simulink model "two_mass_sys"  (R2013b)
settings: Solver=ode45  StartTime=0.0  StopTime=10.0  RelTol=1e-3
undefined symbols (not defined in the file): Cw, JL, Jm, Ks
libraries: powerlib x1
settings Model: Creator=User  LastModifiedBy=User

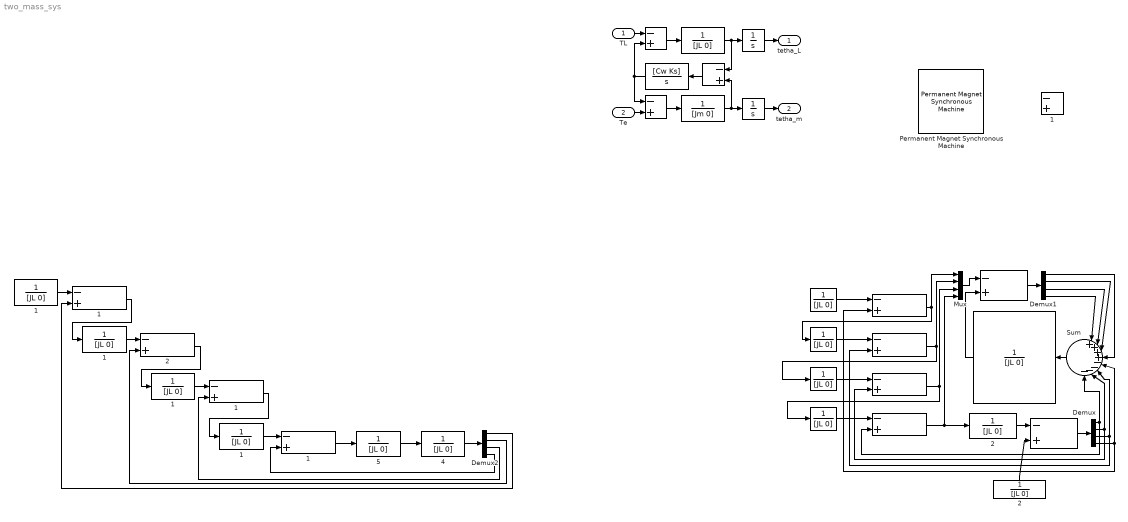
== system two_mass_sys ==
  TL : Inport
  Te : Inport  Port=2
  " " : TransferFcn  Numerator=[Cw Ks]  Denominator=[1 0]
    {,2,4..5} (4 alike) : TransferFcn  Denominator=[JL 0]
  "   " : TransferFcn  Denominator=[Jm 0]
  "    " : Integrator
  "     " : Integrator
  "       " : TransferFcn  Denominator=[JL 0]
  "        " : Sum  Inputs=-+
  "         " : Sum  Inputs=-+
  "           " : Sum  Inputs=-+
  "            " : Sum  Inputs=-+
  "              " : TransferFcn  Denominator=[JL 0]
  "                " : Sum  Inputs=-+
  "                      " : TransferFcn  Denominator=[JL 0]
  "                        " : Sum  Inputs=-+
  "                                " : Sum  Inputs=-+
  "                                  " : TransferFcn  Denominator=[JL 0]
  "                                                                       " : Sum  Inputs=-+
  "                                                                             " : TransferFcn  Denominator=[JL 0]
  "                                                                                 " : Sum  Inputs=-+
  "                                  1" : TransferFcn  Denominator=[JL 0]
  "                                1" : Sum  Inputs=-+
  "                        1" : Sum  Inputs=-+
  "                      1" : TransferFcn  Denominator=[JL 0]
  "              1" : TransferFcn  Denominator=[JL 0]
  "              2" : TransferFcn  Denominator=[JL 0]
  "            2" : Sum  Inputs=-+
  "           1" : Sum  Inputs=-+
  "         1" : Sum  Inputs=-+
  "       1" : TransferFcn  Denominator=[JL 0]
  Demux : Demux
  Demux1 : Demux
  Demux2 : Demux
  Mux : Mux
  Permanent Magnet Synchronous Machine : powerlib/Machines/Permanent Magnet Synchronous Machine  NbPhases=3  FluxDistribution=Sinusoidal  RotorType=Round  MechanicalLoad=Torque Tm  PresetModel=No  ShowDetailedParameters=on  Resistance=0.18  Inductance=8.5e-3  dqInductances=[8.5e-3,8.5e-3]  La=0.000835  MachineConstant=Flux linkage established by magnets (V.s)  Flux=0.07145  VoltageCst=51.8384  TorqueCst=0.4287  Flat=120  Mechanical=[0.00062 0.0003035 4 0]  PolePairs=4  InitialConditions=[0,0, 0,0]  InitialConditions5ph=[0 0 0 0 0 0]  TsPowergui=0  TsBlock=-1  RefAngle=90 degrees behind phase A axis (modified Park)
  Sum : Sum  Inputs=|++++----
  "tetha_L " : Outport
  "tetha_m  " : Outport  Port=2
  wires:
  "  "/1 -> "                "/1, "     "/1
  "     "/1 -> "tetha_L "/1
  "   "/1 -> "                "/2, "    "/1
  "    "/1 -> "tetha_m  "/1
  "         "/1 -> "  "/1
  "        "/1 -> "   "/1
  Te/1 -> "        "/2
  TL/1 -> "         "/1
  " "/1 -> "         "/2, "        "/1
  "                "/1 -> " "/1
  "              "/1 -> "           "/1
  "       "/1 -> "            "/1
  "                      "/1 -> "                        "/1
  "                                  "/1 -> "                                "/1
  "                                "/1 -> "  2"/1, Mux/4
  "                                                                                 "/1 -> Demux1/1
  Sum/1 -> "                                                                             "/1
  Demux1/4 -> Sum/1
  Demux1/3 -> Sum/2
  Demux1/2 -> Sum/3
  Demux1/1 -> Sum/4
  "  4"/1 -> Demux2/1
  "              1"/1 -> "           1"/1
  "           1"/1 -> "       1"/1
  "       1"/1 -> "            2"/1
  "                      1"/1 -> "                        1"/1
  "                                  1"/1 -> "                                1"/1
  "            2"/1 -> "                      1"/1
  "                        1"/1 -> "                                  1"/1
  "                                1"/1 -> "  5"/1
  "  5"/1 -> "  4"/1
  Demux2/4 -> "                                1"/2
  Demux2/3 -> "                        1"/2
  Demux2/2 -> "            2"/2
  Demux2/1 -> "           1"/2
  "                                                                       "/1 -> Demux/1
  "  2"/1 -> "                                                                       "/1
  Mux/1 -> "                                                                                 "/1
  "           "/1 -> "       "/1, Mux/1
  "            "/1 -> "                      "/1, Mux/2
  "                        "/1 -> "                                  "/1, Mux/3
  "                                                                             "/1 -> "                                                                                 "/2
  Demux/1 -> "                                "/2, Sum/8
  Demux/2 -> "                        "/2, Sum/7
  Demux/3 -> "            "/2, Sum/6
  Demux/4 -> "           "/2, Sum/5
  "              2"/1 -> "                                                                       "/2
